simulink model "b_Observer_Design_Sim"  (R2018b)
settings: Solver=VariableStepAuto  StartTime=0.0  StopTime=10.0  RelTol=1e-3
values from neighbouring files (symbols this model uses):
  Initial_Values = [0.01 0.01 0.06 0.2 0.1 0.3]    [c_Observer_Design.m]
  K = 2.98e-06    [a_Initial.m]    (also in c_Observer_Design.m = place(A_Reform, B_Reform, poles))
  L = 0.225    [a_Initial.m]    (also in c_Observer_Design.m = L')
undefined symbols (not defined in the file or in its folder): A_Reform, B_Reform, C_Reform, D_Reform
settings Model: Creator=Milad  LastModifiedBy=Milad
settings DataIOCC: ReturnWorkspaceOutputs=on

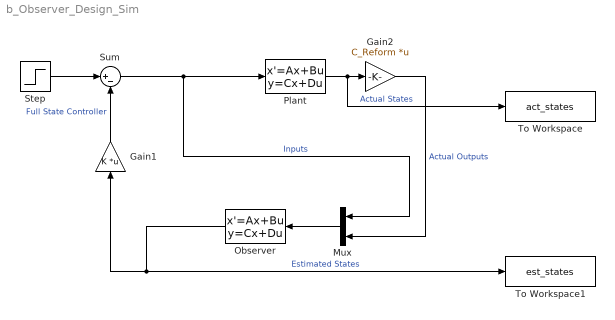
== system b_Observer_Design_Sim ==
  Gain1 : Gain  Gain=K  Multiplication=Matrix(K*u)
  Gain2 : Gain  Gain=C_Reform  Multiplication=Matrix(K*u)
  Mux : Mux  Inputs=2
  Observer : StateSpace  A=A_Reform-L*C_Reform  B=[B_Reform L]  C=eye(6)  D=zeros(6, 9)  InitialCondition=0
  Plant : StateSpace  A=A_Reform  B=B_Reform  C=eye(6)  D=D_Reform  InitialCondition=Initial_Values
  Step : Step  After=0  SampleTime=0
  Sum : Sum  Inputs=|+-
  To Workspace : ToWorkspace  VariableName=act_states  SampleTime=-1
  To Workspace1 : ToWorkspace  VariableName=est_states  SampleTime=-1
  wires:
  Mux/1 -> Observer/1
  Observer/1 -> To Workspace1/1, Gain1/1  "Estimated States"
  Step/1 -> Sum/1
  Plant/1 -> To Workspace/1, Gain2/1  "Actual States"
  Gain1/1 -> Sum/2  "Full State Controller"
  Gain2/1 -> Mux/2  "Actual Outputs"
  Sum/1 -> Mux/1, Plant/1  "Inputs"
